simulink model "force"  (R2019a)
settings: Solver=FixedStepAuto  StartTime=0.0  StopTime=2  FixedStep=1e-3  MaxStep=1e-3  RelTol=1e-3
values from neighbouring files (symbols this model uses):
  f_eff = 2.6*10^(-5)    (= 2.6e-05)    [Untitled3.m]
  Jeff = double(Jeff_c(1))    [Untitled3.m]
undefined symbols (not defined in the file or in its folder): KD, KI, KP, n
settings Model: Creator=sensei  LastModifiedBy=JanAriel

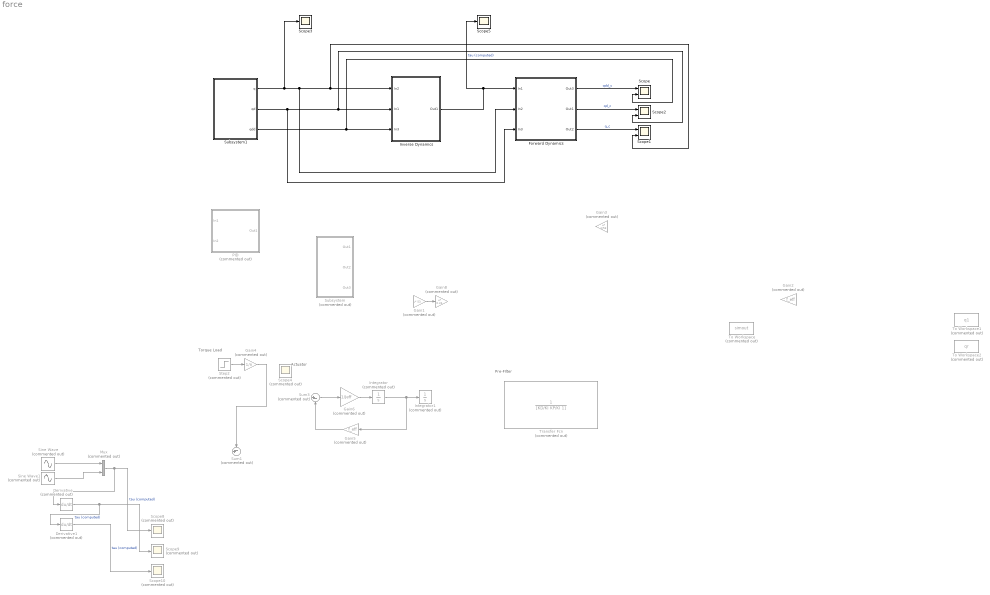
== system force ==
  note: Pre-FIlter
  note: Torque Load
  note: Actuator
  Derivative : Derivative  Commented=on
  Derivative1 : Derivative  Commented=on
  Forward Dynamics : Subsystem
  Gain1 : Gain  Commented=on  Gain=53  Multiplication=Matrix(u*K)
  Gain2 : Gain  Commented=on  Gain=f_eff
  Gain3 : Gain  Commented=on  Gain=1/53  Multiplication=Matrix(u*K)
  Gain4 : Gain  Commented=on  Gain=1/n
  Gain5 : Gain  Commented=on  Gain=f_eff
  Gain6 : Gain  Commented=on  Gain=1/Jeff
  Gain8 : Gain  Commented=on  Gain=0.24  Multiplication=Matrix(u*K)
  Integrator : Integrator  Commented=on
  Integrator1 : Integrator  Commented=on
  Inverse Dynamics : Subsystem
  Mux : Mux  Commented=on  Inputs=2
  PID : Subsystem  Commented=on
  Scope : Scope  NumInputPorts=2
  Scope1 : Scope  NumInputPorts=2
  Scope{4,8..10} (4 alike) : Scope  Commented=on
  Scope2 : Scope  NumInputPorts=2
  Scope3 : Scope
  Scope5 : Scope
  Sine Wave : Sin  Commented=on  SampleTime=0
  Sine Wave1 : Sin  Commented=on  SampleTime=0
  Step2 : Step  Commented=on  Time=5  After=6  SampleTime=0
  Subsystem : Subsystem  Commented=on
  Subsystem1 : Subsystem
  Sum1 : Sum  Commented=on  Inputs=-+|
  Sum3 : Sum  Commented=on  Inputs=|+-
  To Workspace : ToWorkspace  Commented=on  VariableName=simout  SaveFormat=Structure With Time  SampleTime=-1
  To Workspace1 : ToWorkspace  Commented=on  VariableName=q1  SaveFormat=Structure With Time  SampleTime=-1
  To Workspace2 : ToWorkspace  Commented=on  VariableName=qr  SaveFormat=Structure With Time  SampleTime=-1
  Transfer Fcn : TransferFcn  Commented=on  Denominator=[KD/KI KP/KI 1]
  wires:
  Step2/1 -> Gain4/1
  Gain4/1 -> Sum1/1
  Gain5/1 -> Sum3/2
  Gain6/1 -> Integrator/1
  Integrator/1 -> Integrator1/1, Gain5/1
  Sum3/1 -> Gain6/1
  Sine Wave/1 -> Mux/1
  Sine Wave1/1 -> Mux/2
  Derivative/1 -> Scope9/1, Derivative1/1  "tau (computed)"
  Derivative1/1 -> Scope10/1  "tau (computed)"
  Mux/1 -> Scope8/1, Derivative/1  "tau (computed)"
  Gain1/1 -> Gain8/1
  Forward Dynamics/1(Out3) -> Scope/1  "qdd_c"
  Forward Dynamics/2(Out1) -> Scope2/1  "qd_c"
  Forward Dynamics/3(Out2) -> Scope1/1  "q_c"
  Inverse Dynamics/1(Out1) -> Scope5/1, Forward Dynamics/1(In1)  "tau (computed)"
  Subsystem1/1(q) -> Scope3/1, Inverse Dynamics/1(In2), Scope1/2, Forward Dynamics/2(In2)
  Subsystem1/2(qd) -> Inverse Dynamics/2(In1), Scope2/2, Forward Dynamics/3(In3)
  Subsystem1/3(qdd) -> Scope/2, Inverse Dynamics/3(In3)

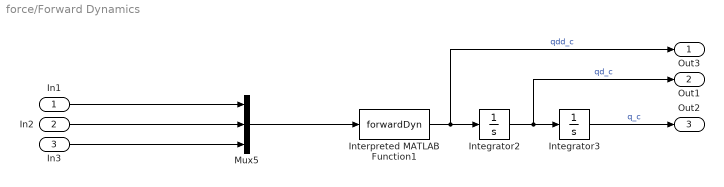
== system force/Forward Dynamics ==
  In1 : Inport
  In2 : Inport  Port=2
  In3 : Inport  Port=3
  Integrator2 : Integrator
  Integrator3 : Integrator
  Interpreted MATLAB Function1 : MATLABFcn  MATLABFcn=forwardDyn  Output1D=off
  Mux5 : Mux  Inputs=3
  Out3 : Outport
  Out1 : Outport  Port=2
  Out2 : Outport  Port=3
  wires:
  In2/1 -> Mux5/2
  In1/1 -> Mux5/1
  Integrator2/1 -> Out1/1, Integrator3/1  "qd_c"
  In3/1 -> Mux5/3
  Integrator3/1 -> Out2/1  "q_c"
  Interpreted MATLAB Function1/1 -> Out3/1, Integrator2/1  "qdd_c"
  Mux5/1 -> Interpreted MATLAB Function1/1

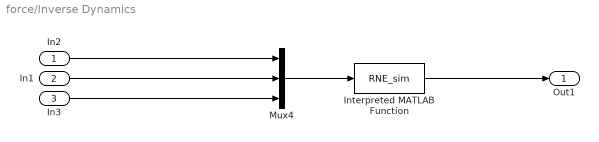
== system force/Inverse Dynamics ==
  In2 : Inport
  In1 : Inport  Port=2
  In3 : Inport  Port=3
  Interpreted MATLAB Function : MATLABFcn  MATLABFcn=RNE_sim  Output1D=off
  Mux4 : Mux  Inputs=3
  Out1 : Outport
  wires:
  In1/1 -> Mux4/2
  Mux4/1 -> Interpreted MATLAB Function/1
  Interpreted MATLAB Function/1 -> Out1/1
  In3/1 -> Mux4/3
  In2/1 -> Mux4/1

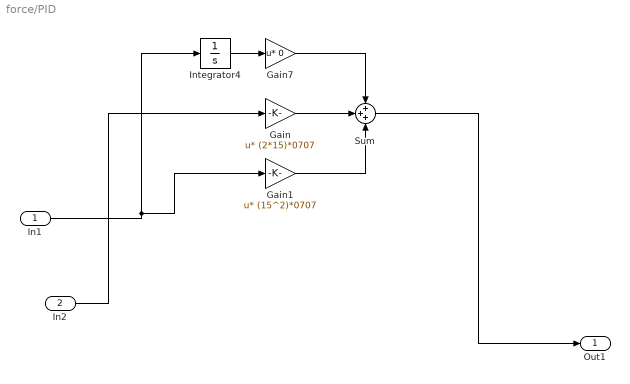
== system force/PID ==
  In1 : Inport
  In2 : Inport  Port=2
  Gain : Gain  Gain=(2*15)*0707  Multiplication=Matrix(u*K)
  Gain1 : Gain  Gain=(15^2)*0707  Multiplication=Matrix(u*K)
  Gain7 : Gain  Gain=0  Multiplication=Matrix(u*K)
  Integrator4 : Integrator
  Sum : Sum  Inputs=+++
  Out1 : Outport
  wires:
  Gain/1 -> Sum/2
  Gain7/1 -> Sum/1
  Sum/1 -> Out1/1
  Gain1/1 -> Sum/3
  In1/1 -> Integrator4/1, Gain1/1
  Integrator4/1 -> Gain7/1
  In2/1 -> Gain/1

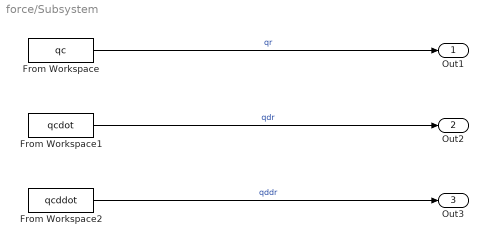
== system force/Subsystem ==
  From Workspace : FromWorkspace  VariableName=qc  SampleTime=0
  From Workspace1 : FromWorkspace  VariableName=qcdot  SampleTime=0
  From Workspace2 : FromWorkspace  VariableName=qcddot  SampleTime=0
  Out1 : Outport
  Out2 : Outport  Port=2
  Out3 : Outport  Port=3
  wires:
  From Workspace1/1 -> Out2/1  "qdr"
  From Workspace2/1 -> Out3/1  "qddr"
  From Workspace/1 -> Out1/1  "qr"

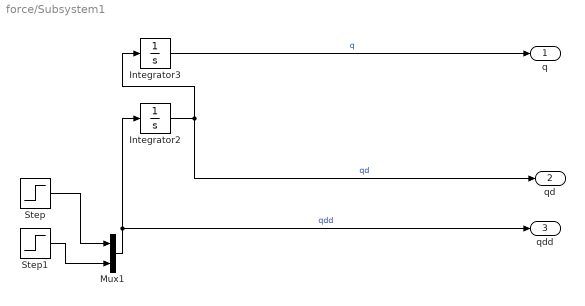
== system force/Subsystem1 ==
  Integrator2 : Integrator
  Integrator3 : Integrator
  Mux1 : Mux  Inputs=2
  Step : Step  SampleTime=0
  Step1 : Step  SampleTime=0
  q : Outport
  qd : Outport  Port=2
  qdd : Outport  Port=3
  wires:
  Step1/1 -> Mux1/2
  Integrator2/1 -> qd/1, Integrator3/1  "qd"
  Mux1/1 -> qdd/1, Integrator2/1  "qdd"
  Step/1 -> Mux1/1
  Integrator3/1 -> q/1  "q"
